simulink model "twelve_pulse_diode_rectifier"  (R2018a)
settings: Solver=VariableStepAuto  StartTime=0.0  StopTime=10.0  RelTol=1e-3
undefined symbols (not defined in the file): D1, Delta
libraries: powerlib x21
settings Model: Creator=Gulten  LastModifiedBy=Gulten

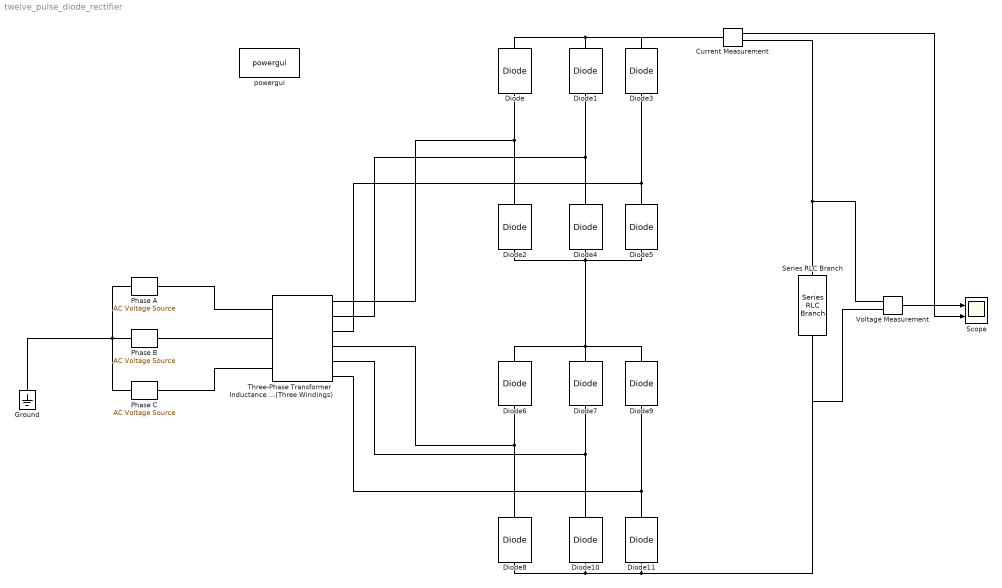
== system twelve_pulse_diode_rectifier ==
  Current Measurement : powerlib/Measurements/Current Measurement  PhasorSimulation=off  OutputType=Complex  PSBequivalent=0
  Diode{,1..11} (12 alike) : powerlib/Power Electronics/Diode  Ron=0.001  Lon=0  Vf=0.8  IC=0  UseSnubber=0  Rs=500  Cs=250e-9  Measurements=off
  Ground : powerlib/Elements/Ground  LConnTagsString=a
  Phase A : powerlib/Electrical Sources/AC Voltage Source  Amplitude=326.6  Phase=0  Frequency=50  SampleTime=0  Measurements=None  BusType=swing  Pref=10e3  Qref=0  Qmin=-inf  Qmax=+inf
  Phase B : powerlib/Electrical Sources/AC Voltage Source  Amplitude=326.6  Phase=240  Frequency=50  SampleTime=0  Measurements=None  BusType=swing  Pref=10e3  Qref=0  Qmin=-inf  Qmax=+inf
  Phase C : powerlib/Electrical Sources/AC Voltage Source  Amplitude=326.6  Phase=120  Frequency=50  SampleTime=0  Measurements=None  BusType=swing  Pref=10e3  Qref=0  Qmin=-inf  Qmax=+inf
  Scope : Scope  NumInputPorts=2
  Series RLC Branch : powerlib/Elements/Series RLC Branch  LConnTagsString=__new0  RConnTagsString=__new0  BranchType=R  Resistance=10  Inductance=1e-3  SetiL0=off  InitialCurrent=0  Capacitance=1e-6  Setx0=off  InitialVoltage=0  Measurements=None
  Three-Phase Transformer Inductance Matrix Type (Three Windings) : powerlib/Elements/Three-Phase Transformer Inductance Matrix Type (Three Windings)  CoreType=Three-limb or five-limb core  Winding1Connection=Delta (D1)  Winding2Connection=Y  Winding3Connection=Delta (D1)  AutoTransformer=off  Measurements=None  NominalPower="[260e6,  60]"  VLLnom="[315e3,  120e3,  43e3]"  WindingResistances="[0.005,  0.005, 0.005]"  NoLoadIexcPos=0.06  NoLoadPlossPos=260e6*0.04/100  ShortCircuitReactancePos="[0.087,  0.166,  0.067]"  ShortCircuitReactancePosAuto="[0.087,  0.166,  0.067]"  NoLoadIexcZero=100  NoLoadPlossZero=260e6*1/100  ShortCircuitReactanceZero=[0.1, 0.2, 0.3 ]  ShortCircuitReactanceZeroAuto=[0.1, 0.2, 0.3 ]  X12ZeroMeasuredWithW3Delta=off
      settings: SourceProductName=Simscape Power Systems  SourceProductBaseCode=PS
  Voltage Measurement : powerlib/Measurements/Voltage Measurement  PhasorSimulation=off  OutputType=Complex  PSBequivalent=0
  powergui : powerlib/powergui  Priority=1  SimulationMode=Continuous  SampleTime=50e-6  frequency=60  Iterations=50  frequencyindice=60  Pbase=100e6  ErrMax=1e-4  UnitsV=kV  UnitsW=MW  buscounter=0  FunctionMessages=off  echomessages=off  EnableUseOfTLC=off  CurrentSourceSwitches=off  DisableSnubberDevices=off  DisableRonSwitches=off  DisableVfSwitches=off  DisplayEquations=off  SolverType=Tustin/Backward Euler (TBE)  Interpol=off  ExternalGateDelay=off  methode=off  Ts=100  x0status=blocks  SPID=on  SwTol=0  HookPort=off  RestoreLinks=warning  ResistiveCurrentMeasurement=off  Frange=[0:2:500]  Ylog=off  Xlog=on  ShowGrid=off  save=off  variable=ZData  structure=0  ZoomFFT=off  StartTime=0.0  cycles=1  DisplayStyle=1  fundamental=60  FreqAxis=off  MaxFrequency=1000  frequencyindicesteady=1  RmsSteady=1  display=off
  wires:
  Voltage Measurement/1 -> Scope/1
  Current Measurement/1 -> Scope/2
  connections:
  Diode/RConn1 -- Current Measurement/LConn1 -- Diode3/RConn1 -- Diode1/RConn1
  Diode4/RConn1 -- Three-Phase Transformer Inductance Matrix Type (Three Windings)/RConn2 -- Diode1/LConn1
  Diode5/RConn1 -- Three-Phase Transformer Inductance Matrix Type (Three Windings)/RConn3 -- Diode3/LConn1
  Diode2/RConn1 -- Three-Phase Transformer Inductance Matrix Type (Three Windings)/RConn1 -- Diode/LConn1
  Diode8/LConn1 -- Diode10/LConn1 -- Voltage Measurement/LConn2 -- Series RLC Branch/RConn1 -- Diode11/LConn1
  Diode2/LConn1 -- Diode7/RConn1 -- Diode9/RConn1 -- Diode6/RConn1 -- Diode5/LConn1 -- Diode4/LConn1
  Diode11/RConn1 -- Three-Phase Transformer Inductance Matrix Type (Three Windings)/RConn6 -- Diode9/LConn1
  Diode10/RConn1 -- Three-Phase Transformer Inductance Matrix Type (Three Windings)/RConn5 -- Diode7/LConn1
  Diode8/RConn1 -- Three-Phase Transformer Inductance Matrix Type (Three Windings)/RConn4 -- Diode6/LConn1
  Phase A/RConn1 -- Three-Phase Transformer Inductance Matrix Type (Three Windings)/LConn1
  Phase B/RConn1 -- Three-Phase Transformer Inductance Matrix Type (Three Windings)/LConn2
  Three-Phase Transformer Inductance Matrix Type (Three Windings)/LConn3 -- Phase C/RConn1
  Phase C/LConn1 -- Ground/LConn1 -- Phase B/LConn1 -- Phase A/LConn1
  Series RLC Branch/LConn1 -- Voltage Measurement/LConn1 -- Current Measurement/RConn1
